simulink model "Single_Phase_PWM"  (R2021a)
settings: Solver=VariableStepAuto  StartTime=0.0  StopTime=0.5  RelTol=1e-3
settings Model: Creator=tanmoyera  LastModifiedBy=tanmoyera

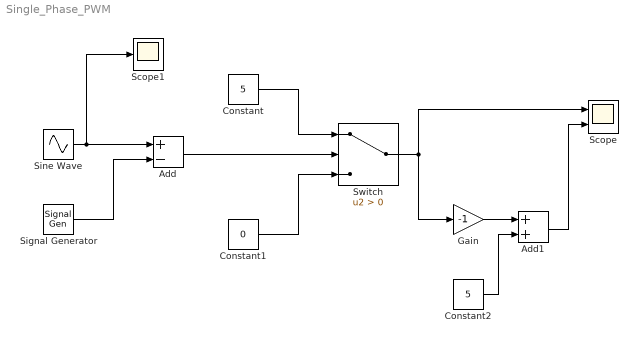
== system Single_Phase_PWM ==
  Add : Sum  Inputs=+-
  Add1 : Sum
  Constant : Constant  Value=5
  Constant1 : Constant  Value=0
  Constant2 : Constant  Value=5
  Gain : Gain  Gain=-1
  Scope : Scope  NumInputPorts=2
  Scope1 : Scope
  Signal Generator : SignalGenerator  Frequency=1000
  Sine Wave : Sin  Amplitude=5  Frequency=314  SampleTime=0
  Switch : Switch  Criteria=u2 > Threshold
  wires:
  Sine Wave/1 -> Scope1/1, Add/1
  Signal Generator/1 -> Add/2
  Add/1 -> Switch/2
  Constant/1 -> Switch/1
  Constant1/1 -> Switch/3
  Switch/1 -> Gain/1, Scope/1
  Gain/1 -> Add1/1
  Constant2/1 -> Add1/2
  Add1/1 -> Scope/2
